simulink model "ship_Track_sin"  (Simulink 10.3)
settings: Solver=ode45  StartTime=0.0  StopTime=1000  RelTol=1e-3  EnableMultiTasking=on
libraries: simulink x2
settings Model: Creator=Administrator  LastModifiedBy=1179956468
settings DataIOCC: LimitDataPoints=on
settings DebuggingCC: SolverPrmCheckMsg=warning
settings ConfigComp: CovSFcnEnable=off

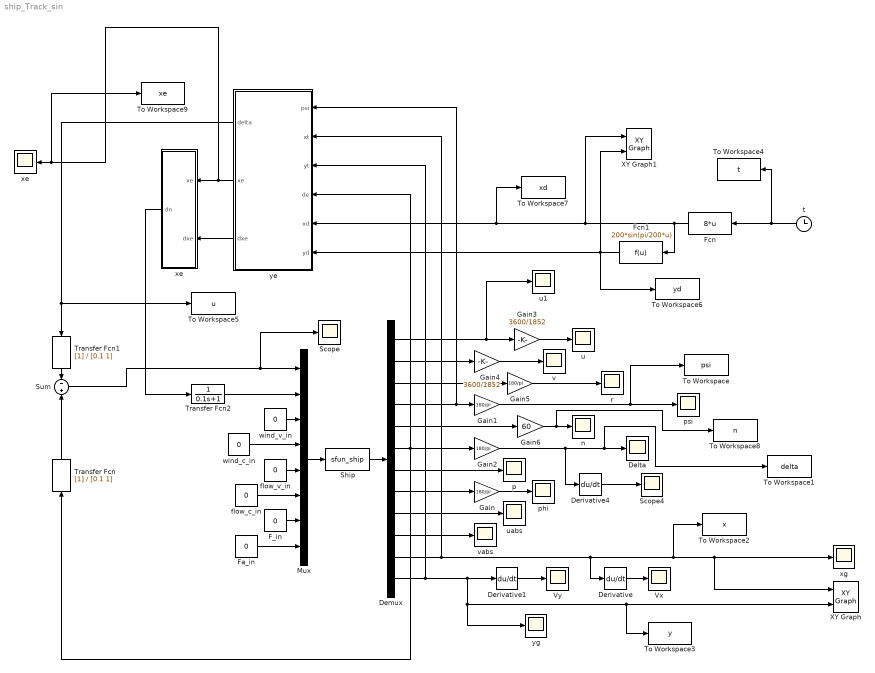
== system ship_Track_sin ==
  Delta : Scope
  Demux : Demux  Outputs=12
  Derivative : Derivative
  Derivative1 : Derivative
  Derivative4 : Derivative
  F_in : Constant  Value=0
  Fa_in : Constant  Value=0
  Fcn : Fcn  Expr=8*u
  Fcn1 : Fcn  Expr=200*sin(pi/200*u)
  Gain{,1..2,5} (4 alike) : Gain  Gain=180/pi
  Gain3 : Gain  Gain=3600/1852
  Gain4 : Gain  Gain=3600/1852
  Gain6 : Gain  Gain=60
  Mux : Mux  Inputs=8
  Scope : Scope
  Scope4 : Scope
  Ship : S-Function  FunctionName=sfun_ship  SFunctionDeploymentMode=off  EnableBusSupport=off
  Sum : Sum  Inputs=-|+
  To Workspace : ToWorkspace  VariableName=psi  SampleTime=-1
  To Workspace1 : ToWorkspace  VariableName=delta  SampleTime=-1
  To Workspace2 : ToWorkspace  VariableName=x  SampleTime=-1
  To Workspace3 : ToWorkspace  VariableName=y  SampleTime=-1
  To Workspace4 : ToWorkspace  VariableName=t  SampleTime=-1
  To Workspace5 : ToWorkspace  VariableName=u  SampleTime=-1
  To Workspace6 : ToWorkspace  VariableName=yd  SampleTime=-1
  To Workspace7 : ToWorkspace  VariableName=xd  SampleTime=-1
  To Workspace8 : ToWorkspace  VariableName=n  SampleTime=-1
  To Workspace9 : ToWorkspace  VariableName=xe  SampleTime=-1
  Transfer Fcn : TransferFcn  Denominator=[0.1 1]
  Transfer Fcn1 : TransferFcn  Denominator=[0.1 1]
  Transfer Fcn2 : TransferFcn  Denominator=[0.1 1]
  "Vx " : Scope
  Vy : Scope
  XY Graph : simulink/Sinks/XY Graph  xmin=0  xmax=2000  ymin=-500  ymax=500  st=-1
  XY Graph1 : simulink/Sinks/XY Graph  xmin=0  xmax=2000  ymin=-500  ymax=500  st=-1
  flow_c_in : Constant  Value=0
  flow_v_in : Constant  Value=0
  n : Scope
  p : Scope
  phi : Scope
  psi : Scope
  r : Scope
  t : Clock
  u : Scope
  u1 : Scope
  uabs : Scope
  v : Scope
  vabs : Scope
  wind_c_in : Constant  Value=0
  wind_v_in : Constant  Value=0
  xe : Scope
  "xe " : Subsystem
  xg : Scope
  ye : Subsystem
  yg : Scope
  wires:
  Ship/1 -> Demux/1
  Demux/1 -> u1/1, Gain3/1
  Demux/2 -> Gain4/1
  Demux/3 -> Gain5/1
  Demux/5 -> Gain6/1
  Demux/6 -> Gain2/1, Transfer Fcn/1, ye/4(de)
  Demux/7 -> p/1
  Demux/8 -> Gain/1
  Gain1/1 -> psi/1, To Workspace/1
  Gain/1 -> phi/1
  Gain3/1 -> u/1
  Gain4/1 -> v/1
  Gain5/1 -> r/1
  Gain6/1 -> To Workspace8/1, n/1
  Demux/9 -> uabs/1
  Demux/10 -> vabs/1
  Demux/12 -> ye/3(yt), Derivative1/1, yg/1, To Workspace3/1, XY Graph/2
  Demux/11 -> ye/2(xt), Derivative/1, To Workspace2/1, XY Graph/1, xg/1
  Derivative/1 -> "Vx "/1
  Derivative1/1 -> Vy/1
  wind_v_in/1 -> Mux/3
  wind_c_in/1 -> Mux/4
  flow_v_in/1 -> Mux/5
  F_in/1 -> Mux/7
  Fa_in/1 -> Mux/8
  flow_c_in/1 -> Mux/6
  Mux/1 -> Ship/1
  Derivative4/1 -> Scope4/1
  ye/1(delta) -> Transfer Fcn1/1, To Workspace5/1
  Demux/4 -> Gain1/1, ye/1(psi)
  Gain2/1 -> Derivative4/1, Delta/1, To Workspace1/1
  Sum/1 -> Mux/1, Scope/1
  Fcn1/1 -> XY Graph1/2, To Workspace6/1, ye/6(yd)
  t/1 -> Fcn/1, To Workspace4/1
  ye/2(xe) -> To Workspace9/1, xe/1, "xe "/1(xe)
  ye/3(dxe) -> "xe "/2(dxe)
  Fcn/1 -> Fcn1/1, ye/5(xd), To Workspace7/1, XY Graph1/1
  "xe "/1(dn) -> Transfer Fcn2/1
  Transfer Fcn/1 -> Sum/2
  Transfer Fcn1/1 -> Sum/1
  Transfer Fcn2/1 -> Mux/2

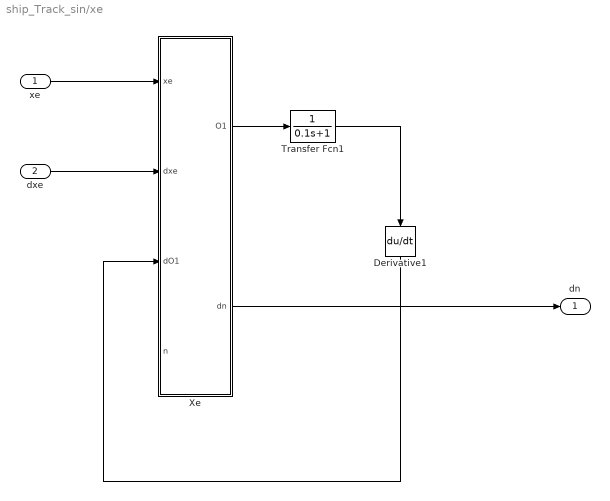
== system ship_Track_sin/xe  ==
  xe : Inport
  dxe : Inport  Port=2
  Derivative1 : Derivative
  Transfer Fcn1 : TransferFcn  Denominator=[0.1 1]
  Xe : MATLAB Function  TreatAsAtomicUnit=on
  dn : Outport
  wires:
  Xe/2(dn) -> dn/1
  xe/1 -> Xe/1(xe)
  Xe/1(O1) -> Transfer Fcn1/1
  Derivative1/1 -> Xe/3(dO1)
  dxe/1 -> Xe/2(dxe)
  Transfer Fcn1/1 -> Derivative1/1

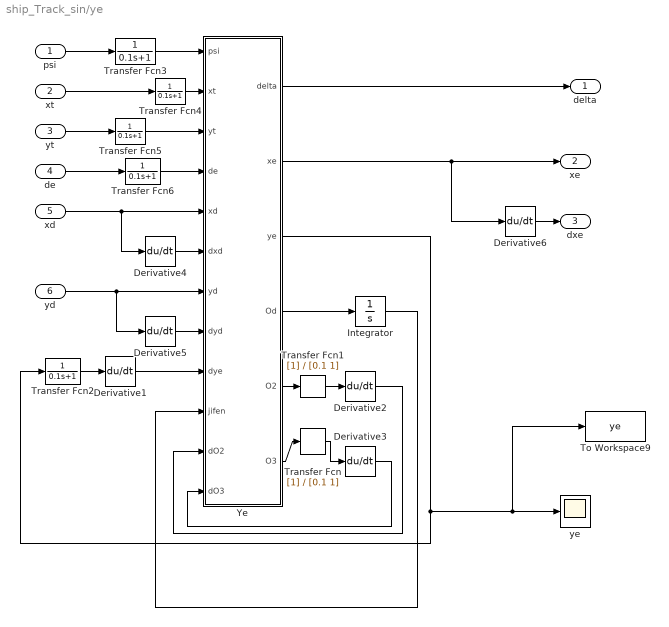
== system ship_Track_sin/ye ==
  psi : Inport
  xt : Inport  Port=2
  yt : Inport  Port=3
  de : Inport  Port=4
  xd : Inport  Port=5
  yd : Inport  Port=6
  Derivative{1..6} (6 alike) : Derivative
  Integrator : Integrator
  To Workspace9 : ToWorkspace  VariableName=ye  SampleTime=-1
  Transfer Fcn{,1..6} (7 alike) : TransferFcn  Denominator=[0.1 1]
  Ye : MATLAB Function  TreatAsAtomicUnit=on
  ye : Scope
  delta : Outport
  xe : Outport  Port=2
  dxe : Outport  Port=3
  wires:
  Ye/6(O3) -> Transfer Fcn/1
  Derivative3/1 -> Ye/12(dO3)
  Ye/5(O2) -> Transfer Fcn1/1
  Derivative2/1 -> Ye/11(dO2)
  Integrator/1 -> Ye/10(jifen)
  Ye/1(delta) -> delta/1
  Ye/4(Od) -> Integrator/1
  psi/1 -> Transfer Fcn3/1
  xt/1 -> Transfer Fcn4/1
  yt/1 -> Transfer Fcn5/1
  Derivative1/1 -> Ye/9(dye)
  Ye/3(ye) -> To Workspace9/1, ye/1, Transfer Fcn2/1
  de/1 -> Transfer Fcn6/1
  xd/1 -> Derivative4/1, Ye/5(xd)
  yd/1 -> Derivative5/1, Ye/7(yd)
  Derivative4/1 -> Ye/6(dxd)
  Derivative5/1 -> Ye/8(dyd)
  Ye/2(xe) -> Derivative6/1, xe/1
  Derivative6/1 -> dxe/1
  Transfer Fcn/1 -> Derivative3/1
  Transfer Fcn1/1 -> Derivative2/1
  Transfer Fcn2/1 -> Derivative1/1
  Transfer Fcn3/1 -> Ye/1(psi)
  Transfer Fcn4/1 -> Ye/2(xt)
  Transfer Fcn5/1 -> Ye/3(yt)
  Transfer Fcn6/1 -> Ye/4(de)

== matlab function xe /Xe ==
  data: xe input double; dxe input double; dO1 input double; O1 output double; dn output double; n input double
function [O1,dn]=fcn(xe,dxe,dO1,n)
K11=0.5;K12=0.5;K13=0.1;K14=0.1;K15=0.1;K16=0;
%K11=0.01;K12=0.5;K13=0.01;K14=0.5;K15=0.000004;K16=0.0001;Tm=4;

O1=K11*tanh(K12*xe)+dxe;
O2=K13*tanh(K14*O1)+dO1;
dn=-K15*O2-K16*tanh(O2);
% nr=n+Tm*dn;

== matlab function ye/Ye ==
  data: psi input double; xt input double; yt input double; de input double; xd input double; dxd input double; yd input double; dyd input double; dye input double; delta output double; xe output double; ye output double; Od output double; O2 output double; O3 output double; jifen input double; dO2 input double; dO3 input double
function [delta,xe,ye,Od,O2,O3] = fcn(psi,xt,yt,de,xd,dxd,yd,dyd,dye,jifen,dO2,dO3)

K0=0.02;K1=1.5;K2=0.02;K3=0.02;K4=10;K5=-160;Te=2.5;
%K0=0.01;K1=0.30;K2=0.05;K3=0.05;K4=1;K5=0.0001;Te=2.5;
 psir=atan2(dyd,dxd);%期望psi(t)
% zitar=atan2((yt-yd),(xt-xd));
% p=sqrt((xt-yd)^2+(yt-xd)^2);
xe=xt-xd;
ye=yt-yd;
%dxe点进模块会看到输出了！！！是将fun的输出xe做微分后输出的，因此不写在这个函数中
% if(de>0)
%     psie=psi-psir-pi/2;
% else
%     psie=psi-psir+pi/2;
% end
 psie=psi-psir;
O1=K1*f(K0*ye)+dye;
Od=f(O1);
O2=psie+K2*jifen;
O3=K3*f(O2)+dO2;
O4=K4*f(O3)+dO3;
%delta=-K5*O4-K6*f(O4);%用舵机模型总是出错
delta=-Te*K5*O4;
 function mean=f(a)
  mean=tanh(a);
%  function mean=f(a)
%  if(a<0.1&&a>-0.1)
%      mean=a;
%  else
%      mean=coth(a)-1/a;
%  end
